simulink model "furuta_pid_option_b_model"  (R2021a)
settings: Solver=VariableStepAuto  StartTime=0.0  StopTime=10  RelTol=1e-3
InitFcn:
  | if ~exist('Kp','var'), load('furuta_pid_model.mat'); end
values from neighbouring files (symbols this model uses):
  Kd = -0.25    [furuta_pid_design.m]    (also in furuta_pid_model.mat; test_run.m = gains(3))
  Ki = -0.8    [furuta_pid_design.m]    (also in furuta_pid_model.mat; test_run.m = gains(2))
  Kp = -2.2    [furuta_pid_design.m]    (also in furuta_pid_model.mat; test_run.m = gains(1))
settings Model: Creator=pankaja  LastModifiedBy=pankaja

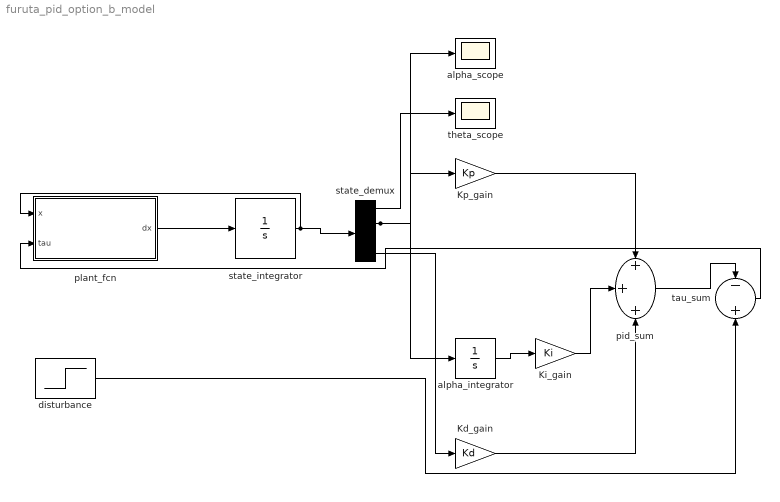
== system furuta_pid_option_b_model ==
  Kd_gain : Gain  Gain=Kd
  Ki_gain : Gain  Gain=Ki
  Kp_gain : Gain  Gain=Kp
  alpha_integrator : Integrator
  alpha_scope : Scope
  disturbance : Step  Time=5  After=0.05  SampleTime=0
  pid_sum : Sum  Inputs=+++
  plant_fcn : MATLAB Function  TreatAsAtomicUnit=on
  state_demux : Demux
  state_integrator : Integrator  InitialCondition=[0; 0.05; 0; 0]
  tau_sum : Sum  Inputs=-+
  theta_scope : Scope
  wires:
  state_integrator/1 -> plant_fcn/1(x), state_demux/1
  tau_sum/1 -> plant_fcn/2(tau)
  plant_fcn/1(dx) -> state_integrator/1
  state_demux/2 -> Kp_gain/1, alpha_integrator/1, alpha_scope/1
  alpha_integrator/1 -> Ki_gain/1
  state_demux/4 -> Kd_gain/1
  Kp_gain/1 -> pid_sum/1
  Ki_gain/1 -> pid_sum/2
  Kd_gain/1 -> pid_sum/3
  pid_sum/1 -> tau_sum/1
  disturbance/1 -> tau_sum/2
  state_demux/1 -> theta_scope/1

== matlab function furuta_pid_option_b_model/plant_fcn ==
  data: x input; dx output; tau input
function dx = plant_fcn(x, tau)
%#codegen
% Nonlinear Furuta pendulum equations of motion.
% x = [theta; alpha; theta_dot; alpha_dot],  tau = motor torque [N*m]
% CAUTION: coefficients must match furuta_params.m.
Jr = 7.86e-5; Mp = 0.024; Lr = 0.085; Lp = 0.0645; Jp = 1.78e-4;
Br = 0.0015; Bp = 0.00005; g = 9.81;
theta = x(1); alpha = x(2); theta_dot = x(3); alpha_dot = x(4);
s = sin(alpha); c = cos(alpha);
M11 = Jr + Mp*Lr^2 + Jp*s^2;
M12 = Mp*Lr*Lp*c;
M22 = Jp;
C1 = 2*Jp*s*c*theta_dot*alpha_dot + Mp*Lr*Lp*s*alpha_dot^2 + Br*theta_dot;
C2 = -Jp*s*c*theta_dot^2 + Bp*alpha_dot - Mp*g*Lp*s;
Mm = [M11 M12; M12 M22];
rhs = [tau - C1; -C2];
acc = Mm\rhs;
dx = [theta_dot; alpha_dot; acc(1); acc(2)];
